simulink model "Askhsh_4"  (R2018b)
settings: Solver=VariableStepAuto  StartTime=0.0  StopTime=4  RelTol=1e-3
libraries: simulink x1
settings Model: Creator=mluser  LastModifiedBy=mluser
settings DataIOCC: ReturnWorkspaceOutputs=on  Refine=10
settings DebuggingCC: UnconnectedInputMsg=none  UnconnectedOutputMsg=none  UnconnectedLineMsg=none
settings ModelReferenceCC: EnableRefExpFcnMdlSchedulingChecks=off
settings RTWCC: Description=Generic Real-Time Target

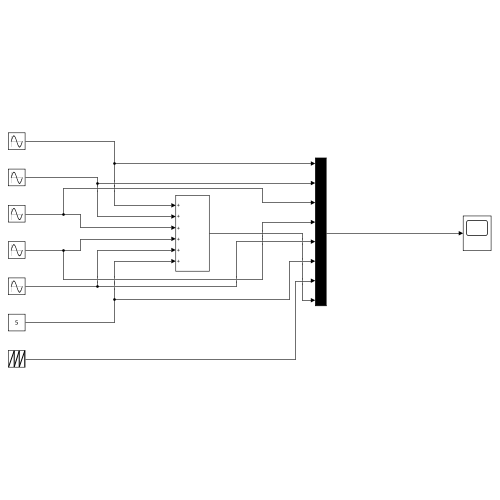
[thumbnail: Simulink's stored preview of the top-level diagram]
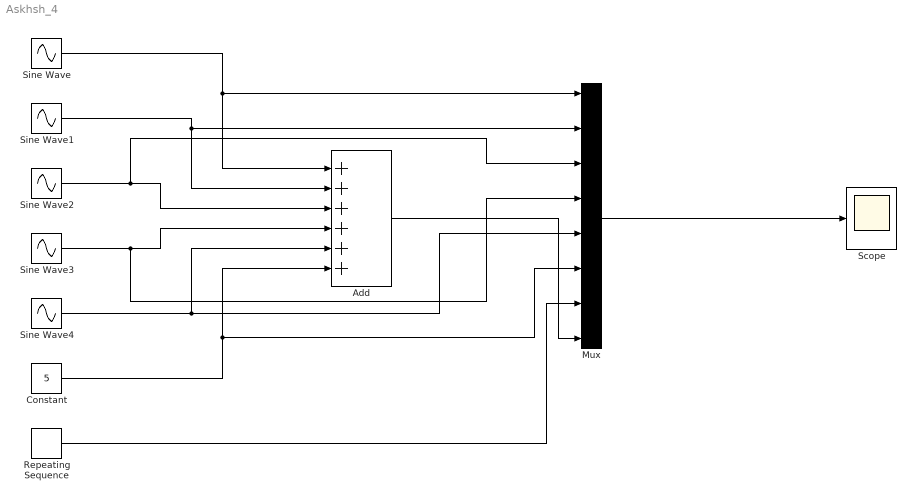
== system Askhsh_4 ==
  Add : Sum  Inputs=++++++
  Constant : Constant  Value=5
  Mux : Mux  Inputs=8
  Repeating Sequence : simulink/Sources/Repeating Sequence  rep_seq_t=[0 2]  rep_seq_y=[0 10]
  Scope : Scope
  Sine Wave : Sin  Amplitude=-10/pi  Frequency=pi  SampleTime=0
  Sine Wave1 : Sin  Amplitude=-10/(2*pi)  Frequency=2*pi  SampleTime=0
  Sine Wave2 : Sin  Amplitude=-10/(3*pi)  Frequency=3*pi  SampleTime=0
  Sine Wave3 : Sin  Amplitude=-10/(4*pi)  Frequency=4*pi  SampleTime=0
  Sine Wave4 : Sin  Amplitude=-10/(5*pi)  Frequency=5*pi  SampleTime=0
  wires:
  Sine Wave1/1 -> Mux/2, Add/2
  Sine Wave2/1 -> Mux/3, Add/3
  Sine Wave3/1 -> Mux/4, Add/4
  Sine Wave4/1 -> Mux/5, Add/5
  Constant/1 -> Mux/6, Add/6
  Sine Wave/1 -> Mux/1, Add/1
  Add/1 -> Mux/8
  Repeating Sequence/1 -> Mux/7
  Mux/1 -> Scope/1
